simulink model "rtwdemo_asap2"  (Simulink 7.6)
settings: Solver=FixedStepDiscrete  StartTime=0.0  StopTime=10.0  RelTol=1e-3
PostLoadFcn:
  | rtwdemo_asap2_data
values from neighbouring files (symbols this model uses):
  k1 = Simulink.Parameter    [rtwdemo_asap2_data.m]
  k2 = Simulink.Parameter    [rtwdemo_asap2_data.m]
  xbreak1 = Simulink.Parameter    [rtwdemo_asap2_data.m]
  xbreak2 = Simulink.Parameter    [rtwdemo_asap2_data.m]
  ybreak = Simulink.Parameter    [rtwdemo_asap2_data.m]
  ydata1 = Simulink.Parameter    [rtwdemo_asap2_data.m]
  ydata2 = Simulink.Parameter    [rtwdemo_asap2_data.m]
  zdata = Simulink.Parameter    [rtwdemo_asap2_data.m]
libraries: rtwdemowidgets x3
Description:
  | Host-Based Data Interface: ASAM-ASAP2 Data Definition File
settings Model: Creator=The MathWorks Inc.  ExtModeAutoUpdateStatusClock=off  TunableVars=K_ExpGlob,K_ExpGlob_FixPt,K_ImpExt,K_ImpExtPt,K_ImpExtPt_FixPt,K_ImpExt_FixPt,K_SimGlob,K_SimGlob_FixPt,XBreak,XBreak_FixPt,YBreak,YBreak_FixPt,YData_ExpGlob,YData_ExpGlob_FixPt,YData_ImpExt,YData_ImpExtPt,YData_ImpExtPt_FixPt,YData_ImpExt_FixPt,YData_SimGlob,YData_SimGlob_FixPt,ZData_ExpGlob,ZData_ExpGlob_FixPt,ZData_ImpExt,ZData_ImpExtPt,ZData_ImpExtPt_FixPt,ZData_ImpExt_FixPt,ZData_SimGlob,ZData_SimGlob_FixPt  TunableVarsStorageClass=ExportedGlobal,ExportedGlobal,ImportedExtern,ImportedExternPointer,ImportedExternPointer,ImportedExtern,Auto,Auto,ExportedGlobal,ExportedGlobal,ExportedGlobal,ExportedGlobal,ExportedGlobal,ExportedGlobal,ImportedExtern,ImportedExternPointer,ImportedExternPointer,ImportedExtern,Auto,Auto,ExportedGlobal,ExportedGlobal,ImportedExtern,ImportedExternPointer,ImportedExternPointer,ImportedExtern,Auto,Auto  TunableVarsTypeQualifier=,,,,,,,,,,,,,,,,,,,,,,,,,,,
settings DataIOCC: SaveOutput=off  SaveTime=off  SignalLoggingName=sigsOut
settings OptimizationCC: InlineParams=on  InlineInvariantSignals=on  StateBitsets=on  DataBitsets=on  UseTempVars=on
settings DebuggingCC: SaveWithParameterizedLinksMsg=none  UnderspecifiedInitializationDetection=Simplified  CheckExecutionContextPreStartOutputMsg=on  CheckExecutionContextRuntimeOutputMsg=on  SolverPrmCheckMsg=none  FcnCallInpInsideContextMsg=Enable All  UniqueDataStoreMsg=error  AssertControl=DisableAll  StrictBusMsg=ErrorOnBusTreatedAsVector
settings HardwareCC: ProdBitPerLong=64  ProdIntDivRoundTo=Zero  ProdEndianess=LittleEndian  ProdWordSize=64  ProdShiftRightIntArith=off  ProdHWDeviceType=Specified
settings RTWCC: TLCOptions=-p0 -aWarnNonSaturatedBlocks=0  GenerateReport=on  RTWVerbose=off  ProcessScript=grt_make_rtw_hook  LaunchReport=on
settings CodeAppCC: ForceParamTrailComments=on
settings GRTTargetCC: GenerateASAP2=on

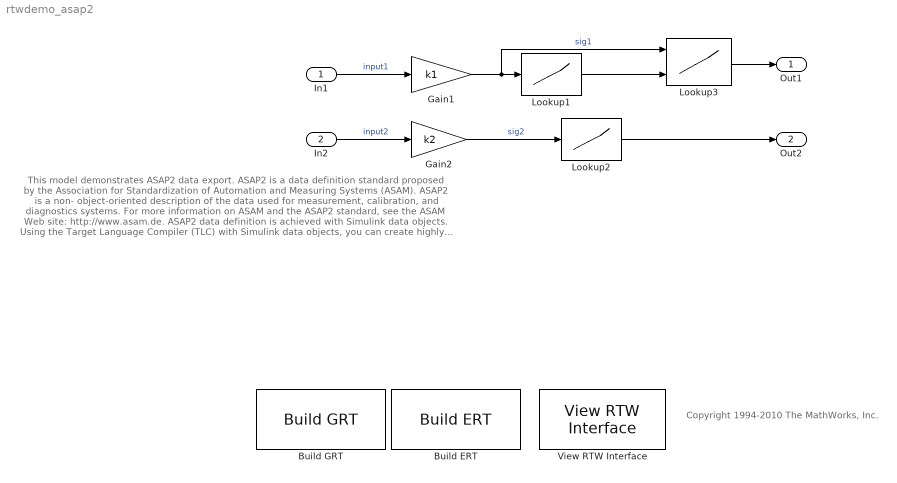
== system rtwdemo_asap2 ==
  note: This model demonstrates ASAP2 data export.  ASAP2 is a data definition standard proposed by the
      | Association for Standardization of Automation and Measuring Systems (ASAM). ASAP2 is a non-
      | object-oriented description of the data used for measurement, calibration, and diagnostics systems.
      | For more information on ASAM and the ASAP2 standard, see the ASAM Web site: http://www.asam.de.
      |
      | ASAP2 data definition is achieved with Simulink data objects.  Using the Target Language Compiler
      | (TLC) with Simulink data objects, you can create highly customized solutions for your application.
      | See the Real-Time Workshop documentation for details on ASAP2 file generation.
      |
      | You configure ASAP2 file generation from the Configuration Parameters Real-Time Workshop
      | Interface page.
  note: Copyright 1994-2010 The MathWorks, Inc.
  In1 : Inport  OutDataTypeStr=double  PortDimensions=1  SampleTime=0.2
  In2 : Inport  Port=2  OutDataTypeStr=int16  PortDimensions=1  SampleTime=0.2
  Build ERT : rtwdemowidgets/Build ERT  SystemSampleTime=-1  attrib_overrides={'GenerateASAP2'}
  Build GRT : rtwdemowidgets/Build GRT  SystemSampleTime=-1  attrib_overrides={'GenerateASAP2'}
  Gain1 : Gain  Gain=k1  OutDataTypeStr=Inherit: Same as input  ParamDataTypeStr=Inherit: Same as input
  Gain2 : Gain  Gain=k2  OutDataTypeStr=Inherit: Same as input  ParamDataTypeStr=Inherit: Same as input
  Lookup1 : Lookup_n-D  NumberOfTableDimensions=1  BreakpointsForDimension1=xbreak1  Table=ydata1  InputSameDT=on
  Lookup2 : Lookup_n-D  NumberOfTableDimensions=1  BreakpointsForDimension1=(-10:1:10)*4  IndexSearchMethod=Evenly spaced points  Table=ydata2  ExtrapMethod=None - Clip  UseLastTableValue=on  RndMeth=Simplest  InputSameDT=on
  Lookup3 : Lookup_n-D  BreakpointsForDimension1=xbreak2  BreakpointsForDimension2=ybreak  Table=zdata  InputSameDT=on
  View RTW Interface : rtwdemowidgets/View RTW Interface  SystemSampleTime=-1
  Out1 : Outport
  Out2 : Outport  Port=2
  wires:
  Gain2/1 -> Lookup2/1  "sig2"
  Gain1/1 -> Lookup1/1, Lookup3/1  "sig1"
  Lookup1/1 -> Lookup3/2
  Lookup3/1 -> Out1/1
  Lookup2/1 -> Out2/1
  In1/1 -> Gain1/1  "input1"
  In2/1 -> Gain2/1  "input2"
